simulink model "A16_3_17_Blockschaltbild"  (R2017b)
settings: Solver=FixedStepDiscrete  StartTime=0.0  StopTime=0.05  FixedStep=Ta  RelTol=1e-3
values from neighbouring files (symbols this model uses):
  a = 0.4    [A16_3_Parameter.m]    (also in A16_4.m)
  A = [exp(-Ta/T1)]    [A16_3_Parameter.m]
  B = [(1-exp(-Ta/T1))*c]    [A16_3_Parameter.m]
  C = [1]    [A16_3_Parameter.m]
  D = 0    [A16_3_Parameter.m]
  Ta = 0.000001    (= 1e-06)    [A16_3_Parameter.m]    (also in A16_4.m)
settings Model: Creator=Bayram  LastModifiedBy=user

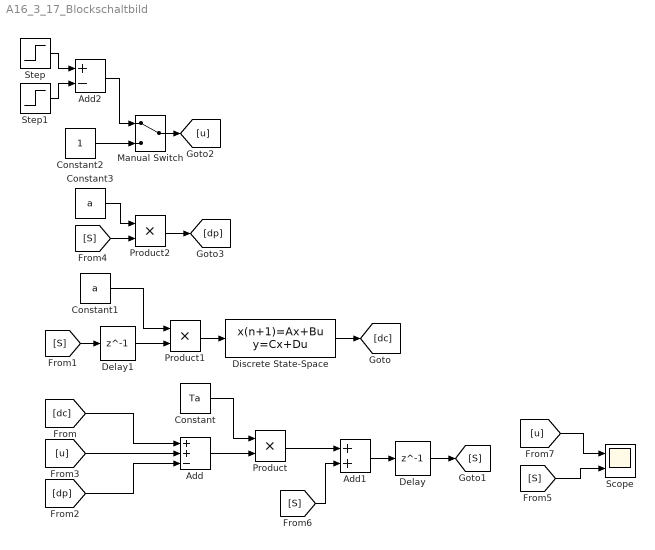
== system A16_3_17_Blockschaltbild ==
  Add : Sum  Inputs=++-
  Add1 : Sum
  Add2 : Sum  Inputs=+-
  Constant : Constant  Value=Ta
  Constant1 : Constant  Value=a
  Constant2 : Constant
  Constant3 : Constant  Value=a
  Delay : Delay  DelayLength=1  InitialCondition=5  UseCircularBuffer=on
  Delay1 : Delay  DelayLength=1  UseCircularBuffer=on
  Discrete State-Space : DiscreteStateSpace  A=A  B=B  C=C  D=D  SampleTime=-1
  Manual Switch : ManualSwitch
  Product : Product
  Product1 : Product
  Product2 : Product
  Scope : Scope  NumInputPorts=2
  Step : Step  Time=10e-3  Before=1  After=1000  SampleTime=0
  Step1 : Step  Time=15e-3  After=999  SampleTime=0
  wires:
  Discrete State-Space/1 -> [dc]
  [S] -> Delay1/1
  Product1/1 -> Discrete State-Space/1
  Constant1/1 -> Product1/1
  Add/1 -> Product/2
  Constant/1 -> Product/1
  [dc] -> Add/1
  [u] -> Add/2
  [dp] -> Add/3
  Product/1 -> Add1/1
  Add1/1 -> Delay/1
  Constant2/1 -> Manual Switch/2
  Product2/1 -> [dp]
  Constant3/1 -> Product2/1
  [S] -> Product2/2
  [S] -> Scope/2
  Delay/1 -> [S]
  [S] -> Add1/2
  Delay1/1 -> Product1/2
  Manual Switch/1 -> [u]
  Step/1 -> Add2/1
  Step1/1 -> Add2/2
  Add2/1 -> Manual Switch/1
  [u] -> Scope/1
